simulink model "homingLoopPNG_for_adjoint"  (Simulink 7.1)
settings: Solver=ode45  StartTime=0.0  StopTime=TFINAL-0.0001  MaxStep=0.001  RelTol=1e-3
values from neighbouring files (symbols this model uses):
  AT = 3    [linearizedPNG_ini.m]    (also in missdisatnce_adjoint.m; missdistance_homing_loop.m; missdistance_linearized.m; truePNG_ini.m = 0)
  HE = 0*(-30/180*pi)    (= 0)    [linearizedPNG_ini.m]    (also in missdisatnce_adjoint.m = 0.523598775598; missdistance_homing_loop.m; missdistance_linearized.m)
  MAX_ACC = 7    [linearizedPNG_ini.m]    (also in truePNG_ini.m = 0.5)
  Tautopilot = 0    [linearizedPNG_ini.m]    (also in missdisatnce_adjoint.m = 2; missdistance_homing_loop.m = 2; missdistance_linearized.m = 2; truePNG_ini.m = 0.2)
  TFINAL = 10    [linearizedPNG_ini.m]    (also in missdisatnce_adjoint.m = 20)
  VC = VM+VT    (= 140)    [linearizedPNG_ini.m]
  VM = 100    [linearizedPNG_ini.m]    (also in truePNG_ini.m = 0.5)
libraries: simulink x1
settings Model: Creator=LESSONS  LastModifiedBy=LESSONS
settings DebuggingCC: SolverPrmCheckMsg=none

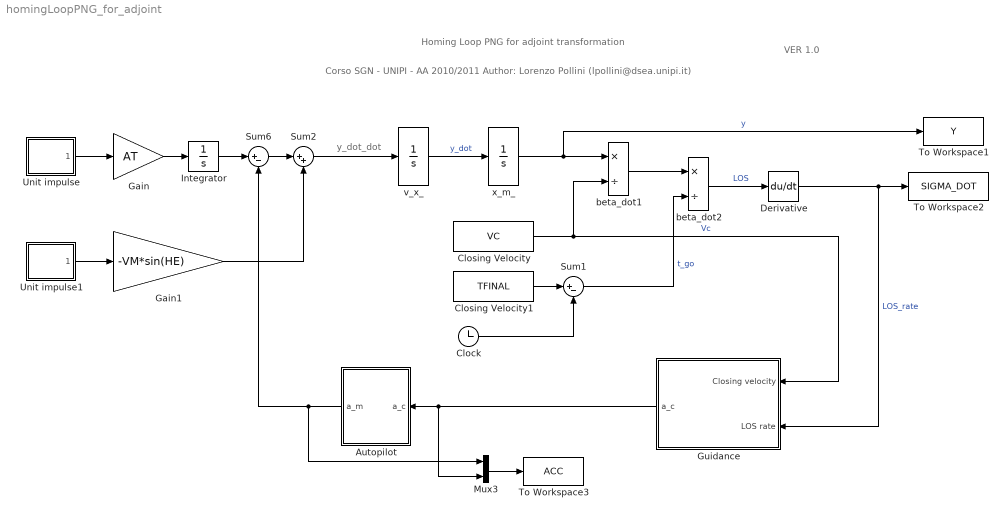
== system homingLoopPNG_for_adjoint ==
  note: y_dot_dot
  note: Homing Loop PNG for adjoint transformation
  note: Corso SGN - UNIPI - AA 2010/2011
      | Author: Lorenzo Pollini (lpollini@dsea.unipi.it)
  note: VER 1.0
  Autopilot : Subsystem  Orientation=left
  Clock : Clock
      settings: Decimation=10
  Closing Velocity : Constant  Value=VC  OutDataType=sfix(16)  OutScaling=2^0
  Closing Velocity1 : Constant  Value=TFINAL  OutDataType=sfix(16)  OutScaling=2^0
  Derivative : Derivative
  Gain : Gain  Gain=AT  ParameterDataType=sfix(16)  ParameterScaling=2^0  OutDataType=sfix(16)  OutScaling=2^0
  Gain1 : Gain  Gain=-VM*sin(HE)  ParameterDataType=sfix(16)  ParameterScaling=2^0  OutDataType=sfix(16)  OutScaling=2^0
  Guidance : Subsystem  Orientation=left
  Integrator : Integrator
  Mux3 : Mux  Inputs=2
  Sum1 : Sum  Inputs=|+-  OutDataType=sfix(16)  OutScaling=2^0
  Sum2 : Sum  Inputs=|++  OutDataType=sfix(16)  OutScaling=2^0
  Sum6 : Sum  Inputs=|+-  OutDataType=sfix(16)  OutScaling=2^0
  To Workspace1 : ToWorkspace  VariableName=Y  SampleTime=-1  SaveFormat=Structure With Time
  To Workspace2 : ToWorkspace  VariableName=SIGMA_DOT  SampleTime=-1  SaveFormat=Structure With Time
  To Workspace3 : ToWorkspace  VariableName=ACC  SampleTime=-1  SaveFormat=Structure With Time
  Unit impulse : Subsystem
  Unit impulse1 : Subsystem
  beta_dot1 : Product  Inputs=*/  OutDataType=sfix(16)  OutScaling=2^-10
  beta_dot2 : Product  Inputs=*/  OutDataType=sfix(16)  OutScaling=2^-10
  v_x_ : Integrator
  x_m_ : Integrator
  wires:
  Integrator/1 -> Sum6/1
  Guidance/1(a_c) -> Autopilot/1(a_c), Mux3/2
  v_x_/1 -> x_m_/1  "y_dot"
  x_m_/1 -> beta_dot1/1, To Workspace1/1  "y"
  beta_dot1/1 -> beta_dot2/1
  Closing Velocity/1 -> beta_dot1/2, Guidance/1(Closing velocity)  "Vc"
  Closing Velocity1/1 -> Sum1/1
  Clock/1 -> Sum1/2
  Sum1/1 -> beta_dot2/2  "t_go"
  beta_dot2/1 -> Derivative/1  "LOS"
  Derivative/1 -> Guidance/2(LOS rate), To Workspace2/1  "LOS_rate"
  Autopilot/1(a_m) -> Sum6/2, Mux3/1
  Gain1/1 -> Sum2/2
  Mux3/1 -> To Workspace3/1
  Unit impulse/1(impulse) -> Gain/1
  Gain/1 -> Integrator/1
  Sum2/1 -> v_x_/1
  Unit impulse1/1(impulse) -> Gain1/1
  Sum6/1 -> Sum2/1

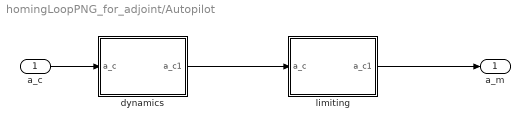
== system homingLoopPNG_for_adjoint/Autopilot ==
  a_c : Inport  OutDataType=sfix(16)  OutScaling=2^0
  dynamics : Subsystem
  limiting : Subsystem
  a_m : Outport  OutDataType=sfix(16)  OutScaling=2^0
  wires:
  a_c/1 -> dynamics/1(a_c)
  dynamics/1(a_c1) -> limiting/1(a_c)
  limiting/1(a_c1) -> a_m/1

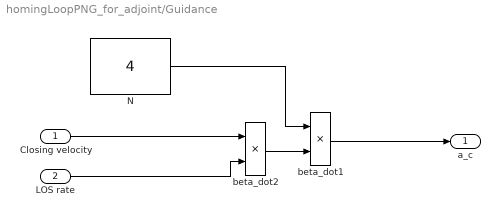
== system homingLoopPNG_for_adjoint/Guidance ==
  Closing velocity : Inport  OutDataType=sfix(16)  OutScaling=2^0
  LOS rate : Inport  Port=2  OutDataType=sfix(16)  OutScaling=2^0
  N : Constant  Value=4  OutDataType=sfix(16)  OutScaling=2^0
  beta_dot1 : Product  Inputs=**  OutDataType=sfix(16)  OutScaling=2^-10
  beta_dot2 : Product  Inputs=**  OutDataType=sfix(16)  OutScaling=2^-10
  a_c : Outport  OutDataType=sfix(16)  OutScaling=2^0
  wires:
  Closing velocity/1 -> beta_dot2/1
  beta_dot1/1 -> a_c/1
  LOS rate/1 -> beta_dot2/2
  beta_dot2/1 -> beta_dot1/2
  N/1 -> beta_dot1/1

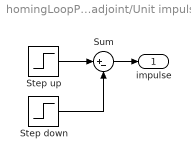
== system homingLoopPNG_for_adjoint/Unit impulse ==
  Step down : Step  Time=eps  After=1/eps  SampleTime=0
  Step up : Step  Time=0  After=1/eps  SampleTime=0
  Sum : Sum  Inputs=|+-  OutDataType=sfix(16)  OutScaling=2^0
  impulse : Outport
  wires:
  Step up/1 -> Sum/1
  Step down/1 -> Sum/2
  Sum/1 -> impulse/1

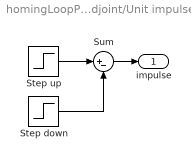
== system homingLoopPNG_for_adjoint/Unit impulse1 ==
  Step down : Step  Time=eps  After=1/eps  SampleTime=0
  Step up : Step  Time=0  After=1/eps  SampleTime=0
  Sum : Sum  Inputs=|+-  OutDataType=sfix(16)  OutScaling=2^0
  impulse : Outport
  wires:
  Sum/1 -> impulse/1
  Step down/1 -> Sum/2
  Step up/1 -> Sum/1

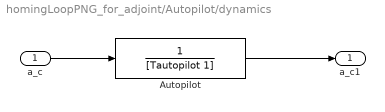
== system homingLoopPNG_for_adjoint/Autopilot/dynamics ==
  a_c : Inport  OutDataType=sfix(16)  OutScaling=2^0
  Autopilot : TransferFcn  Denominator=[Tautopilot 1]
  a_c1 : Outport  OutDataType=sfix(16)  OutScaling=2^0
  wires:
  a_c/1 -> Autopilot/1
  Autopilot/1 -> a_c1/1

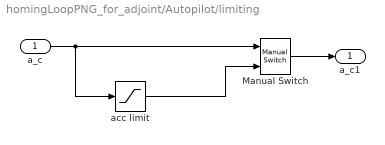
== system homingLoopPNG_for_adjoint/Autopilot/limiting ==
  a_c : Inport  OutDataType=sfix(16)  OutScaling=2^0
  Manual Switch : simulink/Signal Routing/Manual Switch  SystemSampleTime=-1  sw=1  action=0  varsize=off
  acc limit : Saturate  UpperLimit=MAX_ACC  LowerLimit=-MAX_ACC
  a_c1 : Outport  OutDataType=sfix(16)  OutScaling=2^0
  wires:
  Manual Switch/1 -> a_c1/1
  a_c/1 -> Manual Switch/1, acc limit/1
  acc limit/1 -> Manual Switch/2
